simulink model "trafficChart"  (R2016b)
settings: Solver=VariableStepAuto  StartTime=0.0  StopTime=inf  RelTol=1e-3
settings Model: Creator=Radwa  LastModifiedBy=Radwa

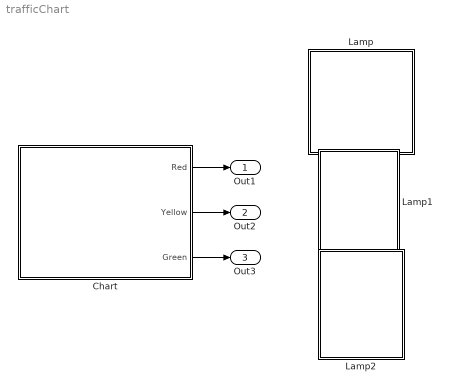
== system trafficChart ==
  Chart : Stateflow chart  TreatAsAtomicUnit=on
  Lamp : Subsystem  DialogController=hmiCreateDDGDialog  IsWebBlock=on  mask(MWDashboardBlock){webBlockId=96de170a-39fc-423e-8846-5a1832b2936f, webBlockType=lamp, ShowInLibBrowser=on, ShowInitialText=on, HMISrcModelName=trafficChart}
      mask prompts: webBlockType "WebBlock Type"; HMISrcModelName "Source Model"
      mask help: SimulinkHMI:dialogs:LampDialogDesc
      mask Help: helpview([docroot '/mapfiles/simulink.map'], 'hmi_lamp')
      mask Display:
      | if strcmp(get_param(bdroot(gcb),'BlockDiagramType'), 'library')
      |     image([(matlabroot) '/toolbox/simulink/hmi/icons/Lamp.png']);
      | end
  Lamp1 : Subsystem  DialogController=hmiCreateDDGDialog  IsWebBlock=on  mask(MWDashboardBlock){webBlockId=1713df2b-0174-45de-ba3e-3c32c142d543, webBlockType=lamp, ShowInLibBrowser=on, ShowInitialText=on, HMISrcModelName=trafficChart}
      mask prompts: webBlockType "WebBlock Type"; HMISrcModelName "Source Model"
      mask help: SimulinkHMI:dialogs:LampDialogDesc
      mask Help: helpview([docroot '/mapfiles/simulink.map'], 'hmi_lamp')
      mask Display:
      | if strcmp(get_param(bdroot(gcb),'BlockDiagramType'), 'library')
      |     image([(matlabroot) '/toolbox/simulink/hmi/icons/Lamp.png']);
      | end
  Lamp2 : Subsystem  DialogController=hmiCreateDDGDialog  IsWebBlock=on  mask(MWDashboardBlock){webBlockId=e03bad0f-0a3c-4ab3-b4b1-010a5f2d1dda, webBlockType=lamp, ShowInLibBrowser=on, ShowInitialText=on, HMISrcModelName=trafficChart}
      mask prompts: webBlockType "WebBlock Type"; HMISrcModelName "Source Model"
      mask help: SimulinkHMI:dialogs:LampDialogDesc
      mask Help: helpview([docroot '/mapfiles/simulink.map'], 'hmi_lamp')
      mask Display:
      | if strcmp(get_param(bdroot(gcb),'BlockDiagramType'), 'library')
      |     image([(matlabroot) '/toolbox/simulink/hmi/icons/Lamp.png']);
      | end
  Out1 : Outport
  Out2 : Outport  Port=2
  Out3 : Outport  Port=3
  wires:
  Chart/1(Red) -> Out1/1
  Chart/2(Yellow) -> Out2/1
  Chart/3(Green) -> Out3/1

== system trafficChart/Lamp ==

== system trafficChart/Lamp1 ==

== system trafficChart/Lamp2 ==

== stateflow chart trafficChart/Chart ==
  state Yellow_Light
    entry:
    Red=0
    Yellow=1;
    Green=0;
  state Green_Light
    entry:
    Red=0;
    Yellow=0;
    Green=1;
  state Red_Light
    entry:
    Red=1;
    Yellow=0;
    Green=0;
  (default) -> Red_Light
  Red_Light -> Yellow_Light : after(10,tick)
  Yellow_Light -> Green_Light : after(5,tick)
  Green_Light -> Red_Light : after(5,tick)
  data: Red output; Yellow output; Green output
